simulink model "AutoThrottle_Guide_100_Env"  (Simulink 8.7)
settings: Solver=FixedStepAuto  StartTime=0.0  StopTime=10.0  RelTol=1e-3
undefined symbols (not defined in the file or in its folder): bias, DiscIntNeverNeededParam
libraries: simulink x1
settings Model: Creator=arnaud  LastModifiedBy=bourbouh
settings DataIOCC: SignalLoggingSaveFormat=ModelDataLogs
settings OptimizationCC: ExpressionDepthLimit=2147483647
settings DebuggingCC: SolverPrmCheckMsg=warning  FcnCallInpInsideContextMsg=UseLocalSettings  StateNameClashWarn=warning
settings GRTTargetCC: GeneratePreprocessorConditionals=Use local settings  CombineOutputUpdateFcns=off  GRTInterface=on

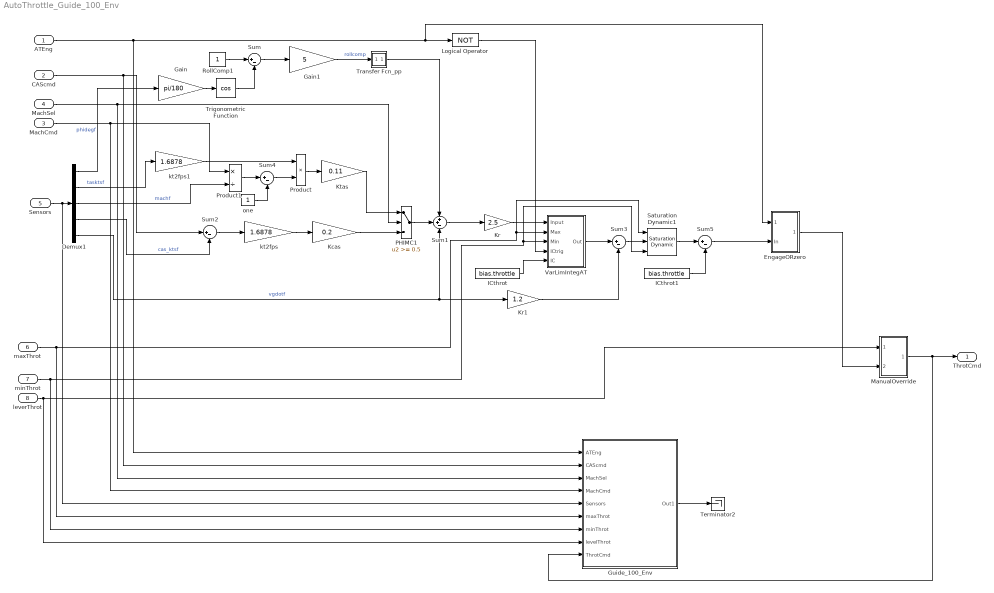
== system AutoThrottle_Guide_100_Env ==
  ATEng : Inport  RequirementInfo={} %GIDa_2f45927d_6c28_4361_8173_5669474b9abd  OutDataTypeStr=boolean
  CAScmd : Inport  RequirementInfo={} %GIDa_92b5701d_5ed6_438c_8e94_843ad865eadf  Port=2
  MachCmd : Inport  RequirementInfo={} %GIDa_c26053c2_6b7f_4bf5_8f7d_768d0d646830  Port=3
  MachSel : Inport  RequirementInfo={} %GIDa_598b16f9_0dbe_4c96_859f_7e96536c1fb2  Port=4
  Sensors : Inport  RequirementInfo={} %GIDa_a55eff7f_fb2b_4f7a_a83b_479b402cff39  Port=5
  maxThrot : Inport  Port=6
  minThrot : Inport  Port=7
  leverThrot : Inport  Port=8
  Demux1 : Demux  Outputs=5
  EngageORzero : Subsystem
  Gain : Gain  RequirementInfo={} %GIDa_44ece66a_e9b1_47ae_9399_459633f82831  Gain=pi/180
  Gain1 : Gain  RequirementInfo={} %GIDa_5f70482a_3c80_415d_8392_528447a4813a  Gain=5
  Guide_100_Env : Subsystem  TreatAsAtomicUnit=on  mask(Observer){AnnotationType=ensures, ObserverType=ellipsoid}
      mask prompts: AnnotationType "Type of annotation (pre/post...)"; ObserverType "Observer type"
      mask help:
      | Set an observer for the system.
      | The annotation type parameter sets the type of observer:
      | - requires : pre-condition
      | - ensures : post-condition
      | - assert : an assertion
      | - observer : the observer computes a special type of properties
      mask TypeOptions AnnotationType: ensures | requires | assert | observer
      mask Callback AnnotationType:
      | paramStr = get_param(gcb, 'MaskValues');
      | 
      | if strcmp(paramStr{1}(1),'o')
      |     set_param(gcb,'MaskVisibilities',{'on';'on'});
      |     paramStr{2} = 'ellipsoid';
      |     set_param(gcb,'MaskValues',paramStr);
      | else
      |     set_param(gcb,'MaskVisibilities',{'on';'off'});
      | end
      mask Callback ObserverType:
      | paramStr = get_param(gcb, 'MaskValues');
      | 
      | if strcmp(paramStr{1}(1),'observer')
      |     set_param(gcb,'MaskVisibilities',{'on';'on'});
      |     paramStr{2} = 'ellipsoid';
      |     set_param(gcb,'MaskValues',paramStr);
      | else
      |     set_param(gcb,'MaskVisibilities',{'on';'off'});
      | end
      mask Display:
      | color('red');
      | text(0.5, 0.5, 'Observer Block', 'horizontalAlignment', 'center');
  ICthrot : Constant  RequirementInfo={} %GIDa_a96462ac_b28c_4fce_82e8_5e3952049bfb  Value=bias.throttle  SampleTime=-1
  ICthrot1 : Constant  RequirementInfo={} %GIDa_23dd534b_a590_436c_b15f_58e24838e8f2  Value=bias.throttle  SampleTime=-1
  Kcas : Gain  RequirementInfo={} %GIDa_1e6984b9_9479_49b0_970a_973f7c32edb7  Gain=0.2
  Kr : Gain  RequirementInfo={} %GIDa_18afb4c5_511e_47fb_85e5_bdfbcffb89de  Gain=2.5
  Kr1 : Gain  RequirementInfo={} %GIDa_9e9297b4_8c75_4533_a8dd_3891075538e5  Gain=1.2
  Ktas : Gain  RequirementInfo={} %GIDa_43c0fedf_b3e4_4e0f_a6fc_568c741b4ee2  Gain=0.11
  Logical Operator : Logic  RequirementInfo={} %GIDa_18e0a705_4fb5_4f14_a12b_8f6e047bc903  Operator=NOT  AllPortsSameDT=off  OutDataTypeStr=boolean
  ManualOverride : Subsystem
  PHIMC1 : Switch  RequirementInfo={} %GIDa_e2112eb0_c2db_4683_9846_bc0eb97a67f4  Threshold=0.5  SaturateOnIntegerOverflow=on
  Product : Product  RequirementInfo={} %GIDa_f2e51a99_89d7_4199_acd2_75b4a5a762fd  RndMeth=Zero
  Product1 : Product  RequirementInfo={} %GIDa_5c94e278_e588_4429_922d_3903b6601868  Inputs=*/  RndMeth=Zero
  RollComp1 : Constant  RequirementInfo={} %GIDa_8f810878_51f3_4d16_a407_aaec8ff4cd8a  SampleTime=-1
  Saturation Dynamic1 : simulink/Discontinuities/Saturation Dynamic  OutMin=[]  OutMax=[]  OutDataTypeStr=Inherit: Same as second input  OutDataType=sfix(16)  OutScaling=2^-10  DoSatur=off
  Sum : Sum  RequirementInfo={} %GIDa_9c88a12f_8eea_40db_a15a_aac24376aa7e  Inputs=|+-
  Sum1 : Sum  RequirementInfo={} %GIDa_fc0b036c_eb6d_4b0a_a40d_b7183183f1bc  Inputs=++-
  Sum2 : Sum  RequirementInfo={} %GIDa_95fcf8e7_99a7_46b3_9e41_77bfb2af0e6e  Inputs=|+-
  Sum3 : Sum  RequirementInfo={} %GIDa_0620e5c6_0d29_4c42_bdd5_2c680788712f  Inputs=|+-
  Sum4 : Sum  RequirementInfo={} %GIDa_a4cfd5ae_8cc7_4a4b_9229_0e28a225e0c7  Inputs=|+-
  Sum5 : Sum  RequirementInfo={} %GIDa_9cd0e9e4_7a0b_4a48_8c2a_57da4ad43678  Inputs=|+-
  Terminator2 : Terminator
  Transfer Fcn_pp : Subsystem  TreatAsAtomicUnit=on
  Trigonometric Function : Trigonometry  RequirementInfo={} %GIDa_82d3b8e2_fba4_4fde_a324_6f5a5fa38b0e  Operator=cos
  VarLimIntegAT : Subsystem  RequirementInfo={} %GIDa_946bbead_442f_495f_943e_e8a8eb5a05a2  TreatAsAtomicUnit=on
  kt2fps : Gain  RequirementInfo={} %GIDa_719dda5c_99e9_4155_8171_b1c9b5878f3a  Gain=1.6878
  kt2fps1 : Gain  RequirementInfo={} %GIDa_b06df2d8_ff63_4d20_83d9_1b3d18a391c7  Gain=1.6878
  one : Constant  RequirementInfo={} %GIDa_79530773_343c_40ed_88d6_a702a3c8b7d7  SampleTime=-1
  ThrotCmd : Outport  RequirementInfo={} %GIDa_10832092_f513_4063_bf4d_710db5c9192f
  wires:
  CAScmd/1 -> Sum2/1, Guide_100_Env/2(CAScmd)
  Sum2/1 -> kt2fps/1
  Sum1/1 -> Kr/1
  kt2fps/1 -> Kcas/1
  Kr/1 -> VarLimIntegAT/1(Input)
  Kr1/1 -> Sum3/2
  Gain1/1 -> Transfer Fcn_pp/1(Inport1)  "rollcomp"
  Sum/1 -> Gain1/1
  Trigonometric Function/1 -> Sum/2
  RollComp1/1 -> Sum/1
  Gain/1 -> Trigonometric Function/1
  Product1/1 -> Sum4/1
  one/1 -> Sum4/2
  Sum4/1 -> Product/2
  kt2fps1/1 -> Product/1
  Product/1 -> Ktas/1
  ICthrot/1 -> VarLimIntegAT/5(IC)
  Sum5/1 -> EngageORzero/2(In)
  ICthrot1/1 -> Sum5/2
  maxThrot/1 -> VarLimIntegAT/2(Max), Saturation Dynamic1/1, Guide_100_Env/6(maxThrot)
  minThrot/1 -> VarLimIntegAT/3(Min), Saturation Dynamic1/3, Guide_100_Env/7(minThrot)
  VarLimIntegAT/1(Out) -> Sum3/1
  Sum3/1 -> Saturation Dynamic1/2
  Saturation Dynamic1/1 -> Sum5/1
  PHIMC1/1 -> Sum1/2
  Kcas/1 -> PHIMC1/3
  Ktas/1 -> PHIMC1/1
  Transfer Fcn_pp/1(Outport1) -> Sum1/1
  Logical Operator/1 -> VarLimIntegAT/4(ICtrig)
  ATEng/1 -> EngageORzero/1(Engage), Logical Operator/1, Guide_100_Env/1(ATEng)
  MachSel/1 -> PHIMC1/2, Guide_100_Env/3(MachSel)
  MachCmd/1 -> Product1/1, Guide_100_Env/4(MachCmd)
  leverThrot/1 -> ManualOverride/1(Man), Guide_100_Env/8(levelThrot)
  ManualOverride/1(Out) -> Guide_100_Env/9(ThrotCmd), ThrotCmd/1
  EngageORzero/1(Out) -> ManualOverride/2(Auto)
  Sensors/1 -> Demux1/1, Guide_100_Env/5(Sensors)
  Demux1/1 -> Gain/1  "phidegf"
  Demux1/2 -> kt2fps1/1  "tasktsf"
  Demux1/3 -> Product1/2  "machf"
  Demux1/4 -> Sum2/2  "cas_ktsf"
  Demux1/5 -> Sum1/3, Kr1/1  "vgdotf"
  Guide_100_Env/1(Out1) -> Terminator2/1

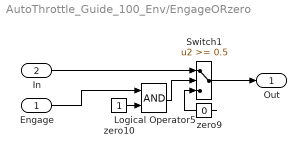
== system AutoThrottle_Guide_100_Env/EngageORzero ==
  Engage : Inport
  In : Inport  Port=2
  Logical Operator5 : Logic  RequirementInfo={} %GIDa_13e72d9c_1630_4494_8181_04ea596767a9  AllPortsSameDT=off  OutDataTypeStr=boolean
  Switch1 : Switch  RequirementInfo={} %GIDa_d89bdcfc_1e33_494f_b3fe_e13e317b4b5d  Threshold=0.5
  zero10 : Constant  RequirementInfo={} %GIDa_d1e784f7_2146_48f6_874a_0add9f175ac2
  zero9 : Constant  RequirementInfo={} %GIDa_df8b3a8b_00d1_4891_87af_e83379ed0682  Value=0
  Out : Outport
  wires:
  Engage/1 -> Logical Operator5/1
  zero10/1 -> Logical Operator5/2
  zero9/1 -> Switch1/3
  In/1 -> Switch1/1
  Logical Operator5/1 -> Switch1/2
  Switch1/1 -> Out/1

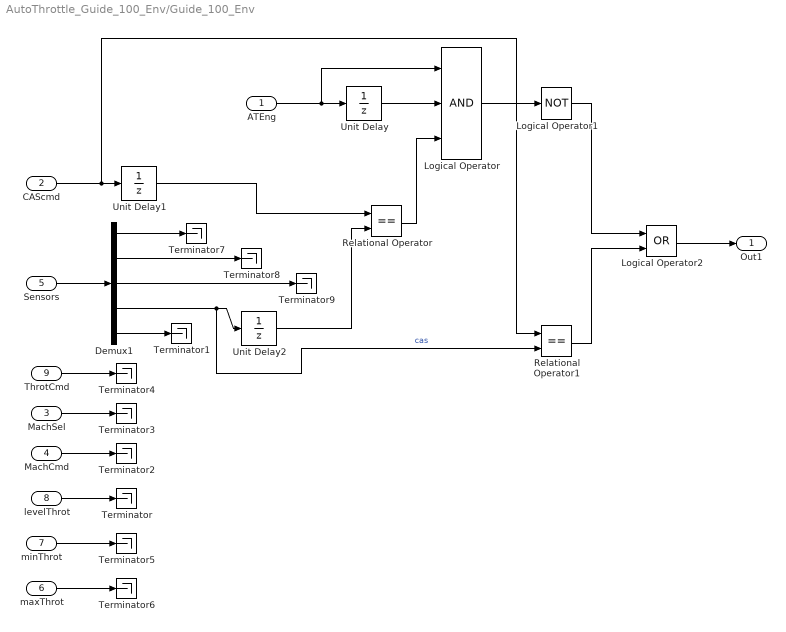
== system AutoThrottle_Guide_100_Env/Guide_100_Env ==
  ATEng : Inport
  CAScmd : Inport  Port=2
  MachSel : Inport  Port=3
  MachCmd : Inport  Port=4
  Sensors : Inport  Port=5
  maxThrot : Inport  Port=6
  minThrot : Inport  Port=7
  levelThrot : Inport  Port=8
  ThrotCmd : Inport  Port=9
  Demux1 : Demux  Outputs=5
  Logical Operator : Logic  Inputs=3  AllPortsSameDT=off  OutDataTypeStr=boolean
  Logical Operator1 : Logic  Operator=NOT  AllPortsSameDT=off  OutDataTypeStr=boolean
  Logical Operator2 : Logic  Operator=OR  AllPortsSameDT=off  OutDataTypeStr=boolean
  Relational Operator : RelationalOperator  Operator===  OutDataTypeStr=boolean
  Relational Operator1 : RelationalOperator  Operator===  OutDataTypeStr=boolean
  Terminator{,1..9} (10 alike) : Terminator
  Unit Delay : UnitDelay  SampleTime=-1
  Unit Delay1 : UnitDelay  SampleTime=-1
  Unit Delay2 : UnitDelay  SampleTime=-1
  Out1 : Outport
  wires:
  levelThrot/1 -> Terminator/1
  MachSel/1 -> Terminator3/1
  MachCmd/1 -> Terminator2/1
  Sensors/1 -> Demux1/1
  minThrot/1 -> Terminator5/1
  maxThrot/1 -> Terminator6/1
  Demux1/4 -> Unit Delay2/1, Relational Operator1/2  "cas"
  Demux1/3 -> Terminator9/1
  Demux1/2 -> Terminator8/1
  Demux1/1 -> Terminator7/1
  Demux1/5 -> Terminator1/1
  ATEng/1 -> Unit Delay/1, Logical Operator/1
  Unit Delay/1 -> Logical Operator/2
  CAScmd/1 -> Unit Delay1/1, Relational Operator1/1
  ThrotCmd/1 -> Terminator4/1
  Unit Delay1/1 -> Relational Operator/1
  Unit Delay2/1 -> Relational Operator/2
  Relational Operator/1 -> Logical Operator/3
  Logical Operator2/1 -> Out1/1
  Logical Operator1/1 -> Logical Operator2/1
  Logical Operator/1 -> Logical Operator1/1
  Relational Operator1/1 -> Logical Operator2/2

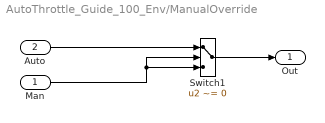
== system AutoThrottle_Guide_100_Env/ManualOverride ==
  Man : Inport
  Auto : Inport  Port=2
  Switch1 : Switch  RequirementInfo={} %GIDa_99412258_89e8_4c84_a7a6_8adb3817b9de  Criteria=u2 ~= 0  Threshold=0.5
  Out : Outport
  wires:
  Man/1 -> Switch1/3, Switch1/2
  Auto/1 -> Switch1/1
  Switch1/1 -> Out/1

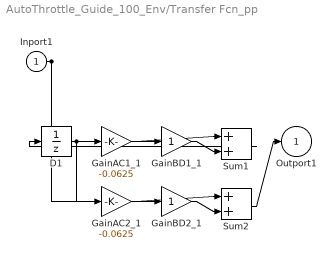
== system AutoThrottle_Guide_100_Env/Transfer Fcn_pp ==
  Inport1 : Inport
  D1 : UnitDelay  SampleTime=-1
  GainAC1_1 : Gain  Gain=-0.0625  SaturateOnIntegerOverflow=on  OutDataTypeStr=Inherit: Same as input  ParamDataTypeStr=Inherit: Same as input
  GainAC2_1 : Gain  Gain=-0.0625  SaturateOnIntegerOverflow=on  OutDataTypeStr=Inherit: Same as input  ParamDataTypeStr=Inherit: Same as input
  GainBD1_1 : Gain  SaturateOnIntegerOverflow=on  OutDataTypeStr=Inherit: Same as input  ParamDataTypeStr=Inherit: Same as input
  GainBD2_1 : Gain  SaturateOnIntegerOverflow=on  OutDataTypeStr=Inherit: Same as input  ParamDataTypeStr=Inherit: Same as input
  Sum1 : Sum  SaturateOnIntegerOverflow=on  InputSameDT=on  OutDataTypeStr=Inherit: Same as first input
  Sum2 : Sum  SaturateOnIntegerOverflow=on  InputSameDT=on  OutDataTypeStr=Inherit: Same as first input
  Outport1 : Outport
  wires:
  D1/1 -> GainAC1_1/1, GainAC2_1/1
  GainAC1_1/1 -> Sum1/1
  GainAC2_1/1 -> Sum2/1
  Inport1/1 -> GainBD1_1/1, GainBD2_1/1
  GainBD1_1/1 -> Sum1/2
  GainBD2_1/1 -> Sum2/2
  Sum1/1 -> D1/1
  Sum2/1 -> Outport1/1

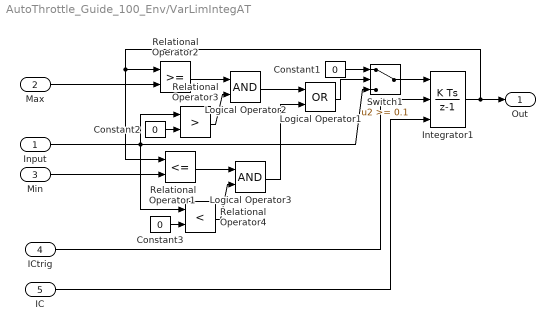
== system AutoThrottle_Guide_100_Env/VarLimIntegAT ==
  Input : Inport  RequirementInfo={} %GIDa_91b38f96_ed38_45a6_8bb9_ff3fb81525df
  Max : Inport  RequirementInfo={} %GIDa_5200ce52_bb44_458c_9945_e382c2e773b4  Port=2
  Min : Inport  RequirementInfo={} %GIDa_600874e9_d5fd_4de5_b948_9284e9d56639  Port=3
  ICtrig : Inport  RequirementInfo={} %GIDa_af678c0a_424b_44b8_aa3a_3f303d846e8e  Port=4
  IC : Inport  RequirementInfo={} %GIDa_872b1a96_8436_4d34_8580_74ad3366301d  Port=5
  Constant1 : Constant  RequirementInfo={} %GIDa_bf704cc0_6bc9_4624_9fa4_e77befe43ee9  Value=0  SampleTime=-1
  Constant2 : Constant  RequirementInfo={} %GIDa_7032ed75_2ad3_41e5_9584_0891c369141c  Value=0  SampleTime=-1
  Constant3 : Constant  RequirementInfo={} %GIDa_f4367f96_4d82_41b7_8e43_0c6cec23a023  Value=0  SampleTime=-1
  Integrator1 : DiscreteIntegrator  ExternalReset=level  InitialConditionSource=external  SampleTime=1.0  ICPrevOutput=DiscIntNeverNeededParam  ICPrevScaledInput=DiscIntNeverNeededParam  mask(DiscretizedDiscreteIntegrator){}
      mask init:
      | %zoh
  Logical Operator1 : Logic  RequirementInfo={} %GIDa_53e2ecf2_1671_4b86_a4e6_7e9f03594f4a  Operator=OR
  Logical Operator2 : Logic  RequirementInfo={} %GIDa_f9639a17_73a7_4a19_b9c3_2b3e1bcf1152
  Logical Operator3 : Logic  RequirementInfo={} %GIDa_53705a9e_f0e6_4df8_b74a_51dda5b71ea0
  Relational Operator1 : RelationalOperator  RequirementInfo={} %GIDa_85cee0a0_d47b_41e2_b8dd_f48b296f5cf4  Operator=<=  InputSameDT=on
  Relational Operator2 : RelationalOperator  RequirementInfo={} %GIDa_74942223_cbc1_42b5_8e5e_e6b9112f9130  InputSameDT=on
  Relational Operator3 : RelationalOperator  RequirementInfo={} %GIDa_ea1202bb_7a42_4314_84fa_c36aa79c966a  Operator=>  InputSameDT=on
  Relational Operator4 : RelationalOperator  RequirementInfo={} %GIDa_c9e3adfb_bd3d_4cfe_9bd6_4a3fd1707fe2  Operator=<  InputSameDT=on
  Switch1 : Switch  RequirementInfo={} %GIDa_ed603307_5c4b_4569_8f05_95ce39b1df88  Threshold=0.1  SaturateOnIntegerOverflow=on  InputSameDT=on
  Out : Outport  RequirementInfo={} %GIDa_a7cb998d_eb28_45ce_8ac9_f1554f32fe4e
  wires:
  IC/1 -> Integrator1/3
  ICtrig/1 -> Integrator1/2
  Min/1 -> Relational Operator1/2
  Max/1 -> Relational Operator2/2
  Constant3/1 -> Relational Operator4/2
  Input/1 -> Switch1/3, Relational Operator3/1, Relational Operator4/1
  Logical Operator3/1 -> Logical Operator1/2
  Relational Operator4/1 -> Logical Operator3/2
  Relational Operator1/1 -> Logical Operator3/1
  Constant2/1 -> Relational Operator3/2
  Logical Operator2/1 -> Logical Operator1/1
  Relational Operator3/1 -> Logical Operator2/2
  Relational Operator2/1 -> Logical Operator2/1
  Logical Operator1/1 -> Switch1/2
  Integrator1/1 -> Relational Operator2/1, Relational Operator1/1, Out/1
  Switch1/1 -> Integrator1/1
  Constant1/1 -> Switch1/1
